simulink model "FDScanningTool"  (R2022b)
settings: Solver=ode1  StartTime=0.0  StopTime=Tobs  FixedStep=delta_t  RelTol=1e-3
values from neighbouring files (symbols this model uses):
  C = 2*pi*Eo*inv(Rp)    [LineParameters.m]    (also in ParametrosAB.m = 2*pi*Epsilon*inv(P); exe_FDScanningTool.m = 0.001)
  delta_t = 10E-6    (= 1e-05)    [exe_FDScanningTool.m]
  dist_time = 1    [exe_FDScanningTool.m]
  dist_value_0 = Idist_value    (= 0.05)    [exe_FDScanningTool.m]
  dist_value_a = [Isignal_dist3(:,1),zeros(samples_window,1)]    [exe_FDScanningTool.m]
  dist_value_b = [Isignal_dist3(:,1),zeros(samples_window,1)]    [exe_FDScanningTool.m]
  dist_value_c = Isignal_dist3    [exe_FDScanningTool.m]
  dist_value_d = Idist_value    (= 0.05)    [exe_FDScanningTool.m]
  dist_value_n = 0.0    (= 0)    [exe_FDScanningTool.m]
  dist_value_p = 0.0    (= 0)    [exe_FDScanningTool.m]
  dist_value_q = 0.0    (= 0)    [exe_FDScanningTool.m]
  f0 = 50    [exe_FDScanningTool.m]    (also in multisine.m = fs/Ns)
  fd = fd0(n)    [exe_FDScanningTool.m]
  Ipeak = 1    [exe_FDScanningTool.m]
  L = 0.001    [exe_FDScanningTool.m]
  phi = (2/3)*pi    (= 2.09439510239)    [exe_FDScanningTool.m]
  R = cond1(:,6)    [LineParameters.m]    (also in exe_FDScanningTool.m = 0.01778)
  R_load = 1E-6    (= 1e-06)    [exe_FDScanningTool.m]
  Rsource = 1E-3    (= 0.001)    [exe_FDScanningTool.m]
  signal_type = 1    [exe_FDScanningTool.m]
  Vpeak = 1    [exe_FDScanningTool.m]
libraries: spsSeriesRLCBranchLib x21, spsControlledCurrentSourceLib x12, spsControlledVoltageSourceLib x12, spsThreePhaseVIMeasurementLib x10, spsThreePhaseSeriesRLCBranchLib x6, spsGroundLib x5, spsDistributedParametersLineFrequencyDependentLib x1, spspowerguiLib x1
(part 2 of 2)

== system FDScanningTool/Frequency Scanner/Current Strategy/Current Fundamental Source/Grid Voltages1 ==
  Constant : Constant  Value=2*pi*f0
  Constant1 : Constant  Value=Ipeak
  Constant3 : Constant  Value=phi
  Constant5 : Constant  Value=phi
  Integrator : Integrator  UpperSaturationLimit=1E100  LowerSaturationLimit=-1E100
  Integrator1 : Integrator  UpperSaturationLimit=1E100  LowerSaturationLimit=-1E100
  Integrator2 : Integrator  UpperSaturationLimit=1E100  LowerSaturationLimit=-1E100
  Product1 : Product
  Product2 : Product
  Product3 : Product
  Sin : Trigonometry  Operator=cos
  Sin1 : Trigonometry  Operator=cos
  Sin2 : Trigonometry  Operator=cos
  Sum1 : Sum  Inputs=|+-
  Sum2 : Sum  Inputs=|++
  VA : Outport
  VB : Outport  Port=2
  VC : Outport  Port=3
  theta : Outport  Port=4
  wires:
  Constant1/1 -> Product1/2, Product2/2, Product3/2
  Sin2/1 -> Product3/1
  Sin/1 -> Product1/1
  Product1/1 -> VA/1
  Sin1/1 -> Product2/1
  Product3/1 -> VC/1
  Product2/1 -> VB/1
  Integrator/1 -> theta/1, Sin/1
  Constant/1 -> Integrator/1, Integrator1/1, Integrator2/1
  Constant5/1 -> Sum2/2
  Sum1/1 -> Sin1/1
  Integrator1/1 -> Sum1/1
  Sum2/1 -> Sin2/1
  Constant3/1 -> Sum1/2
  Integrator2/1 -> Sum2/1

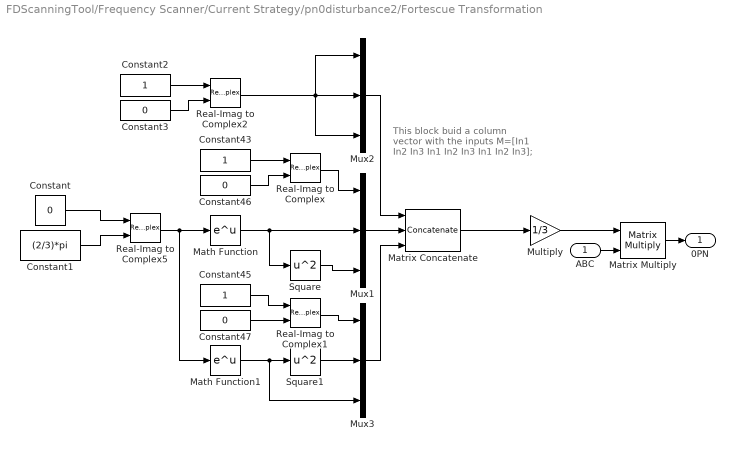
== system FDScanningTool/Frequency Scanner/Current Strategy/pn0disturbance2/Fortescue Transformation ==
  note: This block buid a column vector with the inputs
      | M=[In1 In2 In3
      |       In1 In2 In3
      |       In1 In2 In3];
  ABC : Inport
  Constant{,3,46..47} (4 alike) : Constant  Value=0
  Constant1 : Constant  Value=(2/3)*pi
  Constant2 : Constant
  Constant43 : Constant
  Constant45 : Constant
  Math Function : Math
  Math Function1 : Math
  Matrix Concatenate : Concatenate  NumInputs=3  Mode=Multidimensional array  ConcatenateDimension=2
  Matrix Multiply : Product  Multiplication=Matrix(*)
  Multiply : Gain  Gain=1/3
  Mux1 : Mux  Inputs=3
  Mux2 : Mux  Inputs=3
  Mux3 : Mux  Inputs=3
  Real-Imag to Complex{,1..2,5} (4 alike) : RealImagToComplex
  Square : Math  Operator=square
  Square1 : Math  Operator=square
  0PN : Outport
  wires:
  Square/1 -> Mux1/3
  Math Function/1 -> Mux1/2, Square/1
  Real-Imag to Complex1/1 -> Mux3/1
  Square1/1 -> Mux3/2
  Multiply/1 -> Matrix Multiply/1
  Math Function1/1 -> Square1/1, Mux3/3
  Mux3/1 -> Matrix Concatenate/3
  Constant45/1 -> Real-Imag to Complex1/1
  Matrix Concatenate/1 -> Multiply/1
  Real-Imag to Complex2/1 -> Mux2/2, Mux2/1, Mux2/3
  Real-Imag to Complex5/1 -> Math Function1/1, Math Function/1
  ABC/1 -> Matrix Multiply/2
  Mux2/1 -> Matrix Concatenate/1
  Constant47/1 -> Real-Imag to Complex1/2
  Mux1/1 -> Matrix Concatenate/2
  Real-Imag to Complex/1 -> Mux1/1
  Constant46/1 -> Real-Imag to Complex/2
  Constant43/1 -> Real-Imag to Complex/1
  Matrix Multiply/1 -> 0PN/1
  Constant1/1 -> Real-Imag to Complex5/2
  Constant/1 -> Real-Imag to Complex5/1
  Constant2/1 -> Real-Imag to Complex2/1
  Constant3/1 -> Real-Imag to Complex2/2

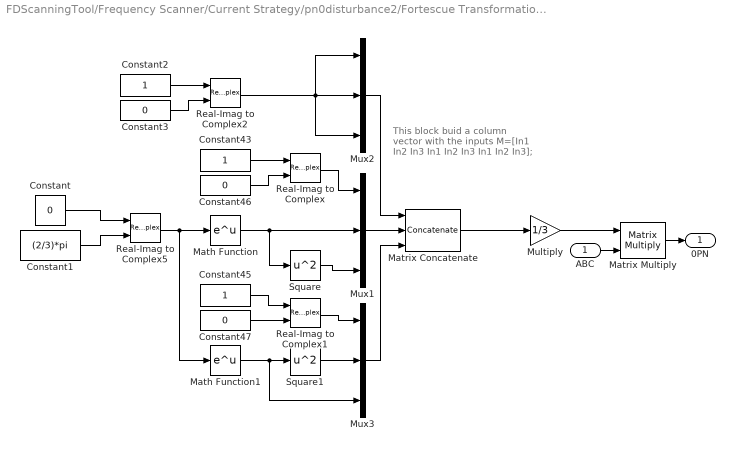
== system FDScanningTool/Frequency Scanner/Current Strategy/pn0disturbance2/Fortescue Transformation1 ==
  note: This block buid a column vector with the inputs
      | M=[In1 In2 In3
      |       In1 In2 In3
      |       In1 In2 In3];
  ABC : Inport
  Constant{,3,46..47} (4 alike) : Constant  Value=0
  Constant1 : Constant  Value=(2/3)*pi
  Constant2 : Constant
  Constant43 : Constant
  Constant45 : Constant
  Math Function : Math
  Math Function1 : Math
  Matrix Concatenate : Concatenate  NumInputs=3  Mode=Multidimensional array  ConcatenateDimension=2
  Matrix Multiply : Product  Multiplication=Matrix(*)
  Multiply : Gain  Gain=1/3
  Mux1 : Mux  Inputs=3
  Mux2 : Mux  Inputs=3
  Mux3 : Mux  Inputs=3
  Real-Imag to Complex{,1..2,5} (4 alike) : RealImagToComplex
  Square : Math  Operator=square
  Square1 : Math  Operator=square
  0PN : Outport
  wires:
  Square/1 -> Mux1/3
  Math Function/1 -> Mux1/2, Square/1
  Real-Imag to Complex1/1 -> Mux3/1
  Square1/1 -> Mux3/2
  Multiply/1 -> Matrix Multiply/1
  Math Function1/1 -> Square1/1, Mux3/3
  Mux3/1 -> Matrix Concatenate/3
  Constant45/1 -> Real-Imag to Complex1/1
  Matrix Concatenate/1 -> Multiply/1
  Real-Imag to Complex2/1 -> Mux2/2, Mux2/1, Mux2/3
  Real-Imag to Complex5/1 -> Math Function1/1, Math Function/1
  ABC/1 -> Matrix Multiply/2
  Mux2/1 -> Matrix Concatenate/1
  Constant47/1 -> Real-Imag to Complex1/2
  Mux1/1 -> Matrix Concatenate/2
  Real-Imag to Complex/1 -> Mux1/1
  Constant46/1 -> Real-Imag to Complex/2
  Constant43/1 -> Real-Imag to Complex/1
  Matrix Multiply/1 -> 0PN/1
  Constant1/1 -> Real-Imag to Complex5/2
  Constant/1 -> Real-Imag to Complex5/1
  Constant2/1 -> Real-Imag to Complex2/1
  Constant3/1 -> Real-Imag to Complex2/2

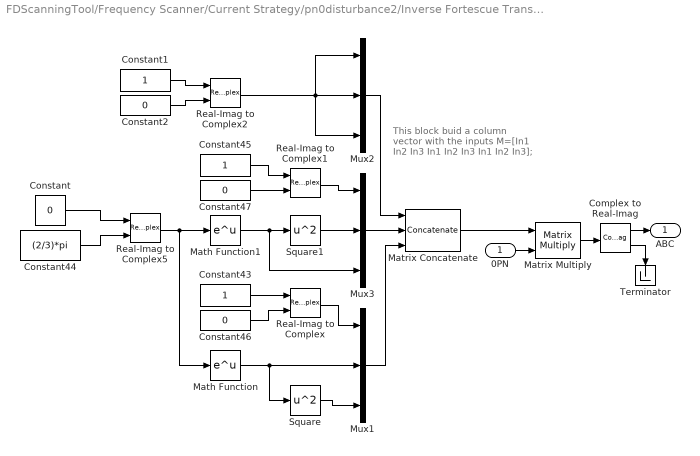
== system FDScanningTool/Frequency Scanner/Current Strategy/pn0disturbance2/Inverse Fortescue Transformation ==
  note: This block buid a column vector with the inputs
      | M=[In1 In2 In3
      |       In1 In2 In3
      |       In1 In2 In3];
  0PN : Inport
  Complex to Real-Imag : ComplexToRealImag
  Constant{,2,46..47} (4 alike) : Constant  Value=0
  Constant1 : Constant
  Constant43 : Constant
  Constant44 : Constant  Value=(2/3)*pi
  Constant45 : Constant
  Math Function : Math
  Math Function1 : Math
  Matrix Concatenate : Concatenate  NumInputs=3  Mode=Multidimensional array  ConcatenateDimension=2
  Matrix Multiply : Product  Multiplication=Matrix(*)
  Mux1 : Mux  Inputs=3
  Mux2 : Mux  Inputs=3
  Mux3 : Mux  Inputs=3
  Real-Imag to Complex{,1..2,5} (4 alike) : RealImagToComplex
  Square : Math  Operator=square
  Square1 : Math  Operator=square
  Terminator : Terminator
  ABC : Outport
  wires:
  Real-Imag to Complex5/1 -> Math Function/1, Math Function1/1
  Constant45/1 -> Real-Imag to Complex1/1
  Constant46/1 -> Real-Imag to Complex/2
  Constant43/1 -> Real-Imag to Complex/1
  Math Function/1 -> Mux1/2, Square/1
  Matrix Concatenate/1 -> Matrix Multiply/1
  Square1/1 -> Mux3/2
  Real-Imag to Complex2/1 -> Mux2/2, Mux2/1, Mux2/3
  0PN/1 -> Matrix Multiply/2
  Math Function1/1 -> Square1/1, Mux3/3
  Constant47/1 -> Real-Imag to Complex1/2
  Mux1/1 -> Matrix Concatenate/3
  Mux2/1 -> Matrix Concatenate/1
  Square/1 -> Mux1/3
  Real-Imag to Complex/1 -> Mux1/1
  Real-Imag to Complex1/1 -> Mux3/1
  Mux3/1 -> Matrix Concatenate/2
  Matrix Multiply/1 -> Complex to Real-Imag/1
  Complex to Real-Imag/1 -> ABC/1
  Complex to Real-Imag/2 -> Terminator/1
  Constant44/1 -> Real-Imag to Complex5/2
  Constant/1 -> Real-Imag to Complex5/1
  Constant2/1 -> Real-Imag to Complex2/2
  Constant1/1 -> Real-Imag to Complex2/1

== system FDScanningTool/Frequency Scanner/Current Strategy/qd0disturbance2/Inverse Park Transform ==
  qd0 : Inport
  theta : Inport  Port=2
  Constant : Constant
  Constant3 : Constant  Value=(2*pi)/3
  Constant4 : Constant  Value=(2*pi)/3
  Cos : Trigonometry  Operator=cos
  Matrix Concatenate : Concatenate  NumInputs=3  Mode=Multidimensional array  ConcatenateDimension=2
  Matrix Multiply : Product  Multiplication=Matrix(*)
  Mux : Mux  Inputs=3
  Mux1 : Mux  Inputs=3
  Sin : Trigonometry
  Sum : Sum  Inputs=+-
  Sum1 : Sum  Inputs=|++
  ABC : Outport
  wires:
  Constant3/1 -> Sum/2
  Constant4/1 -> Sum1/2
  qd0/1 -> Matrix Multiply/2
  Matrix Multiply/1 -> ABC/1
  theta/1 -> Sum1/1, Sum/1, Mux/1
  Sum/1 -> Mux/2
  Sum1/1 -> Mux/3
  Mux/1 -> Sin/1, Cos/1
  Cos/1 -> Matrix Concatenate/1
  Sin/1 -> Matrix Concatenate/2
  Constant/1 -> Mux1/3, Mux1/1, Mux1/2
  Mux1/1 -> Matrix Concatenate/3
  Matrix Concatenate/1 -> Matrix Multiply/1

== system FDScanningTool/Frequency Scanner/Current Strategy/qd0disturbance2/Park Transform ==
  ABC : Inport
  wt : Inport  Port=2
  Constant : Constant  Value=1/2
  Constant1 : Constant  Value=1/2
  Constant2 : Constant  Value=1/2
  Constant3 : Constant  Value=(2*pi)/3
  Constant4 : Constant  Value=(2*pi)/3
  Cos : Trigonometry  Operator=cos
  Cos1 : Trigonometry  Operator=cos
  Cos2 : Trigonometry  Operator=cos
  Gain : Gain  Gain=2/3
  Matrix Concatenate : Concatenate  NumInputs=3  Mode=Multidimensional array  ConcatenateDimension=2
  Matrix Multiply : Product  Multiplication=Matrix(*)
  Mux : Mux  Inputs=3
  Mux1 : Mux  Inputs=3
  Mux2 : Mux  Inputs=3
  Sin : Trigonometry
  Sin1 : Trigonometry
  Sin2 : Trigonometry
  Sum : Sum  Inputs=|+-
  Sum1 : Sum  Inputs=|++
  qd0 : Outport
  wires:
  Sum/1 -> Sin1/1, Cos1/1
  Constant1/1 -> Mux1/3
  Sin2/1 -> Mux2/2
  Gain/1 -> Matrix Multiply/1
  Cos/1 -> Mux/1
  Constant3/1 -> Sum/2
  wt/1 -> Cos/1, Sin/1, Sum/1, Sum1/1
  Sum1/1 -> Sin2/1, Cos2/1
  Mux1/1 -> Matrix Concatenate/2
  Sin/1 -> Mux/2
  Constant4/1 -> Sum1/2
  Constant2/1 -> Mux2/3
  Mux2/1 -> Matrix Concatenate/3
  Cos2/1 -> Mux2/1
  Constant/1 -> Mux/3
  Matrix Concatenate/1 -> Gain/1
  Cos1/1 -> Mux1/1
  Sin1/1 -> Mux1/2
  Mux/1 -> Matrix Concatenate/1
  ABC/1 -> Matrix Multiply/2
  Matrix Multiply/1 -> qd0/1

== system FDScanningTool/Frequency Scanner/Current Strategy/qd0disturbance2/Park Transform1 ==
  ABC : Inport
  wt : Inport  Port=2
  Constant : Constant  Value=1/2
  Constant1 : Constant  Value=1/2
  Constant2 : Constant  Value=1/2
  Constant3 : Constant  Value=(2*pi)/3
  Constant4 : Constant  Value=(2*pi)/3
  Cos : Trigonometry  Operator=cos
  Cos1 : Trigonometry  Operator=cos
  Cos2 : Trigonometry  Operator=cos
  Gain : Gain  Gain=2/3
  Matrix Concatenate : Concatenate  NumInputs=3  Mode=Multidimensional array  ConcatenateDimension=2
  Matrix Multiply : Product  Multiplication=Matrix(*)
  Mux : Mux  Inputs=3
  Mux1 : Mux  Inputs=3
  Mux2 : Mux  Inputs=3
  Sin : Trigonometry
  Sin1 : Trigonometry
  Sin2 : Trigonometry
  Sum : Sum  Inputs=|+-
  Sum1 : Sum  Inputs=|++
  qd0 : Outport
  wires:
  Sum/1 -> Sin1/1, Cos1/1
  Constant1/1 -> Mux1/3
  Sin2/1 -> Mux2/2
  Gain/1 -> Matrix Multiply/1
  Cos/1 -> Mux/1
  Constant3/1 -> Sum/2
  wt/1 -> Cos/1, Sin/1, Sum/1, Sum1/1
  Sum1/1 -> Sin2/1, Cos2/1
  Mux1/1 -> Matrix Concatenate/2
  Sin/1 -> Mux/2
  Constant4/1 -> Sum1/2
  Constant2/1 -> Mux2/3
  Mux2/1 -> Matrix Concatenate/3
  Cos2/1 -> Mux2/1
  Constant/1 -> Mux/3
  Matrix Concatenate/1 -> Gain/1
  Cos1/1 -> Mux1/1
  Sin1/1 -> Mux1/2
  Mux/1 -> Matrix Concatenate/1
  ABC/1 -> Matrix Multiply/2
  Matrix Multiply/1 -> qd0/1

== system FDScanningTool/Frequency Scanner/Voltage Strategy/ABCdisturbance/Multi-tone ==
  Clock : Clock
  Constant1 : Constant  Value=0
  From Workspace : FromWorkspace  VariableName=dist_value_a  SampleTime=delta_t
  From Workspace1 : FromWorkspace  VariableName=dist_value_b  SampleTime=delta_t
  From Workspace2 : FromWorkspace  VariableName=dist_value_c  SampleTime=delta_t
  Mux : Mux  Inputs=3
  Switch1 : Switch  Criteria=u2 > Threshold  Threshold=dist_time  SaturateOnIntegerOverflow=off  InputSameDT=off
  Switch2 : Switch  Criteria=u2 > Threshold  Threshold=dist_time  SaturateOnIntegerOverflow=off  InputSameDT=off
  Switch3 : Switch  Criteria=u2 > Threshold  Threshold=dist_time  SaturateOnIntegerOverflow=off  InputSameDT=off
  ABC : Outport
  wires:
  Switch2/1 -> Mux/2
  From Workspace2/1 -> Switch3/1
  Constant1/1 -> Switch3/3, Switch2/3, Switch1/3
  From Workspace1/1 -> Switch2/1
  Switch3/1 -> Mux/3
  Clock/1 -> Switch1/2, Switch2/2, Switch3/2
  Switch1/1 -> Mux/1
  From Workspace/1 -> Switch1/1
  Mux/1 -> ABC/1

== system FDScanningTool/Frequency Scanner/Voltage Strategy/ABCdisturbance/Single-tone ==
  note: ABC perturbance
  Constant10 : Constant  Value=phi
  Constant12 : Constant  Value=2*pi*fd  SampleTime=delta_t
  Constant9 : Constant  Value=phi
  Integrator5 : Integrator  UpperSaturationLimit=1E100  LowerSaturationLimit=-1E100
  Mux : Mux  Inputs=3
  Product1 : Product
  Product2 : Product
  Product3 : Product
  Sin : Trigonometry  Operator=cos
  Sin1 : Trigonometry  Operator=cos
  Sin2 : Trigonometry  Operator=cos
  Step1 : Step  Time=dist_time  After=dist_value_a  SampleTime=delta_t
  Step2 : Step  Time=dist_time  After=dist_value_b  SampleTime=delta_t
  Step3 : Step  Time=dist_time  After=dist_value_c  SampleTime=delta_t
  Sum6 : Sum  Inputs=|+-
  Sum7 : Sum  Inputs=|++
  ABC : Outport
  wires:
  Sin/1 -> Product1/1
  Sum7/1 -> Sin2/1
  Product1/1 -> Mux/1
  Integrator5/1 -> Sum7/1, Sin/1, Sum6/1
  Sin1/1 -> Product2/1
  Sin2/1 -> Product3/1
  Constant9/1 -> Sum6/2
  Constant10/1 -> Sum7/2
  Step3/1 -> Product3/2
  Step2/1 -> Product2/2
  Constant12/1 -> Integrator5/1
  Sum6/1 -> Sin1/1
  Step1/1 -> Product1/2
  Product2/1 -> Mux/2
  Product3/1 -> Mux/3
  Mux/1 -> ABC/1

== system FDScanningTool/Frequency Scanner/Voltage Strategy/Voltage Fundamental Source/Grid Voltages ==
  Constant : Constant  Value=2*pi*f0
  Constant1 : Constant  Value=Vpeak
  Constant3 : Constant  Value=phi
  Constant5 : Constant  Value=phi
  Integrator : Integrator  UpperSaturationLimit=1E100  LowerSaturationLimit=-1E100
  Integrator1 : Integrator  UpperSaturationLimit=1E100  LowerSaturationLimit=-1E100
  Integrator2 : Integrator  UpperSaturationLimit=1E100  LowerSaturationLimit=-1E100
  Product1 : Product
  Product2 : Product
  Product3 : Product
  Sin : Trigonometry  Operator=cos
  Sin1 : Trigonometry  Operator=cos
  Sin2 : Trigonometry  Operator=cos
  Sum1 : Sum  Inputs=|+-
  Sum2 : Sum  Inputs=|++
  VA : Outport
  VB : Outport  Port=2
  VC : Outport  Port=3
  theta : Outport  Port=4
  wires:
  Constant1/1 -> Product1/2, Product2/2, Product3/2
  Sin2/1 -> Product3/1
  Sin/1 -> Product1/1
  Product1/1 -> VA/1
  Sin1/1 -> Product2/1
  Product3/1 -> VC/1
  Product2/1 -> VB/1
  Integrator/1 -> theta/1, Sin/1
  Constant/1 -> Integrator/1, Integrator1/1, Integrator2/1
  Constant5/1 -> Sum2/2
  Sum1/1 -> Sin1/1
  Integrator1/1 -> Sum1/1
  Sum2/1 -> Sin2/1
  Constant3/1 -> Sum1/2
  Integrator2/1 -> Sum2/1

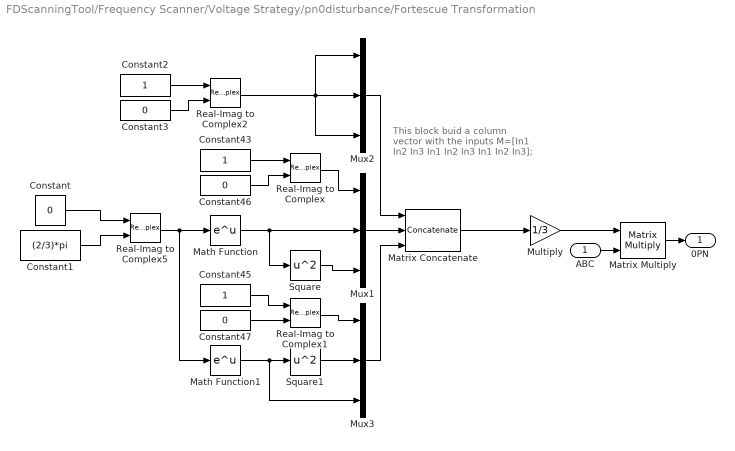
== system FDScanningTool/Frequency Scanner/Voltage Strategy/pn0disturbance/Fortescue Transformation ==
  note: This block buid a column vector with the inputs
      | M=[In1 In2 In3
      |       In1 In2 In3
      |       In1 In2 In3];
  ABC : Inport
  Constant{,3,46..47} (4 alike) : Constant  Value=0
  Constant1 : Constant  Value=(2/3)*pi
  Constant2 : Constant
  Constant43 : Constant
  Constant45 : Constant
  Math Function : Math
  Math Function1 : Math
  Matrix Concatenate : Concatenate  NumInputs=3  Mode=Multidimensional array  ConcatenateDimension=2
  Matrix Multiply : Product  Multiplication=Matrix(*)
  Multiply : Gain  Gain=1/3
  Mux1 : Mux  Inputs=3
  Mux2 : Mux  Inputs=3
  Mux3 : Mux  Inputs=3
  Real-Imag to Complex{,1..2,5} (4 alike) : RealImagToComplex
  Square : Math  Operator=square
  Square1 : Math  Operator=square
  0PN : Outport
  wires:
  Square/1 -> Mux1/3
  Math Function/1 -> Mux1/2, Square/1
  Real-Imag to Complex1/1 -> Mux3/1
  Square1/1 -> Mux3/2
  Multiply/1 -> Matrix Multiply/1
  Math Function1/1 -> Square1/1, Mux3/3
  Mux3/1 -> Matrix Concatenate/3
  Constant45/1 -> Real-Imag to Complex1/1
  Matrix Concatenate/1 -> Multiply/1
  Real-Imag to Complex2/1 -> Mux2/2, Mux2/1, Mux2/3
  Real-Imag to Complex5/1 -> Math Function1/1, Math Function/1
  ABC/1 -> Matrix Multiply/2
  Mux2/1 -> Matrix Concatenate/1
  Constant47/1 -> Real-Imag to Complex1/2
  Mux1/1 -> Matrix Concatenate/2
  Real-Imag to Complex/1 -> Mux1/1
  Constant46/1 -> Real-Imag to Complex/2
  Constant43/1 -> Real-Imag to Complex/1
  Matrix Multiply/1 -> 0PN/1
  Constant1/1 -> Real-Imag to Complex5/2
  Constant/1 -> Real-Imag to Complex5/1
  Constant2/1 -> Real-Imag to Complex2/1
  Constant3/1 -> Real-Imag to Complex2/2

== system FDScanningTool/Frequency Scanner/Voltage Strategy/pn0disturbance/Fortescue Transformation1 ==
  note: This block buid a column vector with the inputs
      | M=[In1 In2 In3
      |       In1 In2 In3
      |       In1 In2 In3];
  ABC : Inport
  Constant{,3,46..47} (4 alike) : Constant  Value=0
  Constant1 : Constant  Value=(2/3)*pi
  Constant2 : Constant
  Constant43 : Constant
  Constant45 : Constant
  Math Function : Math
  Math Function1 : Math
  Matrix Concatenate : Concatenate  NumInputs=3  Mode=Multidimensional array  ConcatenateDimension=2
  Matrix Multiply : Product  Multiplication=Matrix(*)
  Multiply : Gain  Gain=1/3
  Mux1 : Mux  Inputs=3
  Mux2 : Mux  Inputs=3
  Mux3 : Mux  Inputs=3
  Real-Imag to Complex{,1..2,5} (4 alike) : RealImagToComplex
  Square : Math  Operator=square
  Square1 : Math  Operator=square
  0PN : Outport
  wires:
  Square/1 -> Mux1/3
  Math Function/1 -> Mux1/2, Square/1
  Real-Imag to Complex1/1 -> Mux3/1
  Square1/1 -> Mux3/2
  Multiply/1 -> Matrix Multiply/1
  Math Function1/1 -> Square1/1, Mux3/3
  Mux3/1 -> Matrix Concatenate/3
  Constant45/1 -> Real-Imag to Complex1/1
  Matrix Concatenate/1 -> Multiply/1
  Real-Imag to Complex2/1 -> Mux2/2, Mux2/1, Mux2/3
  Real-Imag to Complex5/1 -> Math Function1/1, Math Function/1
  ABC/1 -> Matrix Multiply/2
  Mux2/1 -> Matrix Concatenate/1
  Constant47/1 -> Real-Imag to Complex1/2
  Mux1/1 -> Matrix Concatenate/2
  Real-Imag to Complex/1 -> Mux1/1
  Constant46/1 -> Real-Imag to Complex/2
  Constant43/1 -> Real-Imag to Complex/1
  Matrix Multiply/1 -> 0PN/1
  Constant1/1 -> Real-Imag to Complex5/2
  Constant/1 -> Real-Imag to Complex5/1
  Constant2/1 -> Real-Imag to Complex2/1
  Constant3/1 -> Real-Imag to Complex2/2

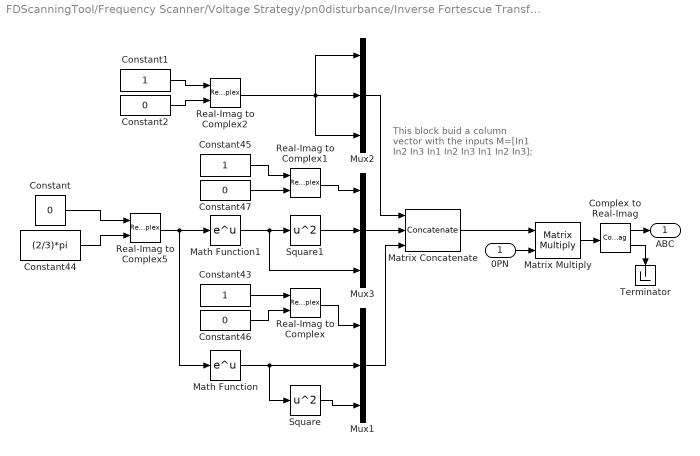
== system FDScanningTool/Frequency Scanner/Voltage Strategy/pn0disturbance/Inverse Fortescue Transformation ==
  note: This block buid a column vector with the inputs
      | M=[In1 In2 In3
      |       In1 In2 In3
      |       In1 In2 In3];
  0PN : Inport
  Complex to Real-Imag : ComplexToRealImag
  Constant{,2,46..47} (4 alike) : Constant  Value=0
  Constant1 : Constant
  Constant43 : Constant
  Constant44 : Constant  Value=(2/3)*pi
  Constant45 : Constant
  Math Function : Math
  Math Function1 : Math
  Matrix Concatenate : Concatenate  NumInputs=3  Mode=Multidimensional array  ConcatenateDimension=2
  Matrix Multiply : Product  Multiplication=Matrix(*)
  Mux1 : Mux  Inputs=3
  Mux2 : Mux  Inputs=3
  Mux3 : Mux  Inputs=3
  Real-Imag to Complex{,1..2,5} (4 alike) : RealImagToComplex
  Square : Math  Operator=square
  Square1 : Math  Operator=square
  Terminator : Terminator
  ABC : Outport
  wires:
  Real-Imag to Complex5/1 -> Math Function/1, Math Function1/1
  Constant45/1 -> Real-Imag to Complex1/1
  Constant46/1 -> Real-Imag to Complex/2
  Constant43/1 -> Real-Imag to Complex/1
  Math Function/1 -> Mux1/2, Square/1
  Matrix Concatenate/1 -> Matrix Multiply/1
  Square1/1 -> Mux3/2
  Real-Imag to Complex2/1 -> Mux2/2, Mux2/1, Mux2/3
  0PN/1 -> Matrix Multiply/2
  Math Function1/1 -> Square1/1, Mux3/3
  Constant47/1 -> Real-Imag to Complex1/2
  Mux1/1 -> Matrix Concatenate/3
  Mux2/1 -> Matrix Concatenate/1
  Square/1 -> Mux1/3
  Real-Imag to Complex/1 -> Mux1/1
  Real-Imag to Complex1/1 -> Mux3/1
  Mux3/1 -> Matrix Concatenate/2
  Matrix Multiply/1 -> Complex to Real-Imag/1
  Complex to Real-Imag/1 -> ABC/1
  Complex to Real-Imag/2 -> Terminator/1
  Constant44/1 -> Real-Imag to Complex5/2
  Constant/1 -> Real-Imag to Complex5/1
  Constant2/1 -> Real-Imag to Complex2/2
  Constant1/1 -> Real-Imag to Complex2/1

== system FDScanningTool/Frequency Scanner/Voltage Strategy/qd0disturbance/Inverse Park Transform ==
  qd0 : Inport
  theta : Inport  Port=2
  Constant : Constant
  Constant3 : Constant  Value=(2*pi)/3
  Constant4 : Constant  Value=(2*pi)/3
  Cos : Trigonometry  Operator=cos
  Matrix Concatenate : Concatenate  NumInputs=3  Mode=Multidimensional array  ConcatenateDimension=2
  Matrix Multiply : Product  Multiplication=Matrix(*)
  Mux : Mux  Inputs=3
  Mux1 : Mux  Inputs=3
  Sin : Trigonometry
  Sum : Sum  Inputs=+-
  Sum1 : Sum  Inputs=|++
  ABC : Outport
  wires:
  Constant3/1 -> Sum/2
  Constant4/1 -> Sum1/2
  qd0/1 -> Matrix Multiply/2
  Matrix Multiply/1 -> ABC/1
  theta/1 -> Sum1/1, Sum/1, Mux/1
  Sum/1 -> Mux/2
  Sum1/1 -> Mux/3
  Mux/1 -> Sin/1, Cos/1
  Cos/1 -> Matrix Concatenate/1
  Sin/1 -> Matrix Concatenate/2
  Constant/1 -> Mux1/3, Mux1/1, Mux1/2
  Mux1/1 -> Matrix Concatenate/3
  Matrix Concatenate/1 -> Matrix Multiply/1

== system FDScanningTool/Frequency Scanner/Voltage Strategy/qd0disturbance/Inverse Park Transform1 ==
  qd0 : Inport
  theta : Inport  Port=2
  Constant : Constant
  Constant3 : Constant  Value=(2*pi)/3
  Constant4 : Constant  Value=(2*pi)/3
  Cos : Trigonometry  Operator=cos
  Matrix Concatenate : Concatenate  NumInputs=3  Mode=Multidimensional array  ConcatenateDimension=2
  Matrix Multiply : Product  Multiplication=Matrix(*)
  Mux : Mux  Inputs=3
  Mux1 : Mux  Inputs=3
  Sin : Trigonometry
  Sum : Sum  Inputs=+-
  Sum1 : Sum  Inputs=|++
  ABC : Outport
  wires:
  Constant3/1 -> Sum/2
  Constant4/1 -> Sum1/2
  qd0/1 -> Matrix Multiply/2
  Matrix Multiply/1 -> ABC/1
  theta/1 -> Sum1/1, Sum/1, Mux/1
  Sum/1 -> Mux/2
  Sum1/1 -> Mux/3
  Mux/1 -> Sin/1, Cos/1
  Cos/1 -> Matrix Concatenate/1
  Sin/1 -> Matrix Concatenate/2
  Constant/1 -> Mux1/3, Mux1/1, Mux1/2
  Mux1/1 -> Matrix Concatenate/3
  Matrix Concatenate/1 -> Matrix Multiply/1

== system FDScanningTool/Frequency Scanner/Voltage Strategy/qd0disturbance/Park Transform ==
  ABC : Inport
  wt : Inport  Port=2
  Constant : Constant  Value=1/2
  Constant1 : Constant  Value=1/2
  Constant2 : Constant  Value=1/2
  Constant3 : Constant  Value=(2*pi)/3
  Constant4 : Constant  Value=(2*pi)/3
  Cos : Trigonometry  Operator=cos
  Cos1 : Trigonometry  Operator=cos
  Cos2 : Trigonometry  Operator=cos
  Gain : Gain  Gain=2/3
  Matrix Concatenate : Concatenate  NumInputs=3  Mode=Multidimensional array  ConcatenateDimension=2
  Matrix Multiply : Product  Multiplication=Matrix(*)
  Mux : Mux  Inputs=3
  Mux1 : Mux  Inputs=3
  Mux2 : Mux  Inputs=3
  Sin : Trigonometry
  Sin1 : Trigonometry
  Sin2 : Trigonometry
  Sum : Sum  Inputs=|+-
  Sum1 : Sum  Inputs=|++
  qd0 : Outport
  wires:
  Sum/1 -> Sin1/1, Cos1/1
  Constant1/1 -> Mux1/3
  Sin2/1 -> Mux2/2
  Gain/1 -> Matrix Multiply/1
  Cos/1 -> Mux/1
  Constant3/1 -> Sum/2
  wt/1 -> Cos/1, Sin/1, Sum/1, Sum1/1
  Sum1/1 -> Sin2/1, Cos2/1
  Mux1/1 -> Matrix Concatenate/2
  Sin/1 -> Mux/2
  Constant4/1 -> Sum1/2
  Constant2/1 -> Mux2/3
  Mux2/1 -> Matrix Concatenate/3
  Cos2/1 -> Mux2/1
  Constant/1 -> Mux/3
  Matrix Concatenate/1 -> Gain/1
  Cos1/1 -> Mux1/1
  Sin1/1 -> Mux1/2
  Mux/1 -> Matrix Concatenate/1
  ABC/1 -> Matrix Multiply/2
  Matrix Multiply/1 -> qd0/1

== system FDScanningTool/Frequency Scanner/Voltage Strategy/qd0disturbance/Park Transform1 ==
  ABC : Inport
  wt : Inport  Port=2
  Constant : Constant  Value=1/2
  Constant1 : Constant  Value=1/2
  Constant2 : Constant  Value=1/2
  Constant3 : Constant  Value=(2*pi)/3
  Constant4 : Constant  Value=(2*pi)/3
  Cos : Trigonometry  Operator=cos
  Cos1 : Trigonometry  Operator=cos
  Cos2 : Trigonometry  Operator=cos
  Gain : Gain  Gain=2/3
  Matrix Concatenate : Concatenate  NumInputs=3  Mode=Multidimensional array  ConcatenateDimension=2
  Matrix Multiply : Product  Multiplication=Matrix(*)
  Mux : Mux  Inputs=3
  Mux1 : Mux  Inputs=3
  Mux2 : Mux  Inputs=3
  Sin : Trigonometry
  Sin1 : Trigonometry
  Sin2 : Trigonometry
  Sum : Sum  Inputs=|+-
  Sum1 : Sum  Inputs=|++
  qd0 : Outport
  wires:
  Sum/1 -> Sin1/1, Cos1/1
  Constant1/1 -> Mux1/3
  Sin2/1 -> Mux2/2
  Gain/1 -> Matrix Multiply/1
  Cos/1 -> Mux/1
  Constant3/1 -> Sum/2
  wt/1 -> Cos/1, Sin/1, Sum/1, Sum1/1
  Sum1/1 -> Sin2/1, Cos2/1
  Mux1/1 -> Matrix Concatenate/2
  Sin/1 -> Mux/2
  Constant4/1 -> Sum1/2
  Constant2/1 -> Mux2/3
  Mux2/1 -> Matrix Concatenate/3
  Cos2/1 -> Mux2/1
  Constant/1 -> Mux/3
  Matrix Concatenate/1 -> Gain/1
  Cos1/1 -> Mux1/1
  Sin1/1 -> Mux1/2
  Mux/1 -> Matrix Concatenate/1
  ABC/1 -> Matrix Multiply/2
  Matrix Multiply/1 -> qd0/1
